simulink library "simulink"  (Simulink 6.0)
settings: Solver=ode45  SolverMode=SingleTasking  StartTime=0.0  StopTime=10.0  RelTol=1e-3
PostLoadFcn:
  | setsysloc(bdroot)
undefined symbols (not defined in the file or in its folder): DiscIntNeverNeededParam, getdatatypespecs, NumBits1, NumBits2, sfunxy, sigbuilder_block, slcm, Slope1, Slope2
libraries: simulink x82, eml_lib x1
(part 3 of 5)

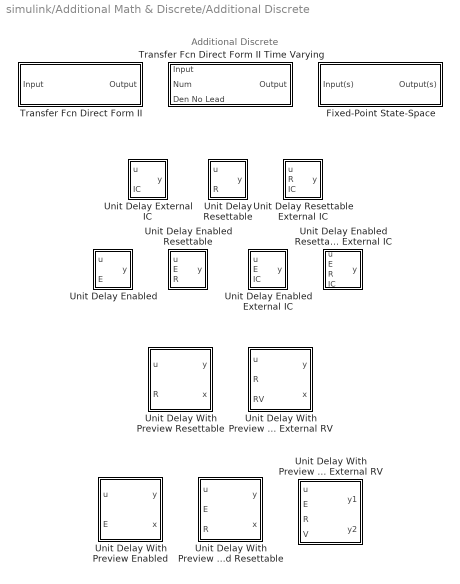
== system simulink/Additional Math & Discrete/Additional Discrete ==
  note: Additional Discrete
  Fixed-Point State-Space : Subsystem  mask(Fixed-Point State-Space){A=[2.6020 -2.2793 0.6708; 1 0 0; 0 1 0], B=[ 1; 0; 0], C=[0.0184    0.0024    0.0055], D=[0.0033], X0=0.0, InternalDataType=float('double'), StateEqScaling=2^0, OutputEqScaling=2^0, LockScale=off, RndMeth=Floor, DoSatur=off}
      mask prompts: A "State Matrix A:"; B "Input Matrix B:"; C "Output Matrix C:"; D "Direct Feedthrough Matrix D:"; X0 "Initial condition for state:"; InternalDataType "Data type for internal calculations:     ex.  sfix(16),  uint(8),  float('single')"; StateEqScaling "Scaling for State Equation AX+BU:   ex.  2^-9"; OutputEqScaling "Scaling for Output Equation CX+DU:   ex.  2^-9"; LockScale "Lock output scaling so autoscaling tool can't change it"; RndMeth "Round toward:"; DoSatur "Saturate to max or min when overflows occur"
      mask help: Discrete-time State-Space Realization
      mask init:
      | blkH = gcbh;
      | blkName = getfullname(blkH);
      | 
      | vRndMeth = get_param(blkH,'RndMeth');
      | vDoSatur = get_param(blkH,'DoSatur');
      | blks = {'State Matrix A','Input Matrix B','Output Matrix C','Direct Link Matrix D','Sum Output Equation','Sum State Equation','Downcast Next State X','Downcast Output Y'};
      | for i = 1:length(blks)
      |   set_param([blkName,'/',blks{i}],'RndMeth',vRndMeth, ...
      | 	  'DoSatur',vDoSatur);
      | end
      mask StyleString: edit,edit,edit,edit,edit,edit,edit,edit,checkbox,popup(Zero|Nearest|Ceiling|Floor),checkbox
      mask TabNameString: Main,Main,Main,Main,Main,Signal data types,Signal data types,Signal data types,Signal data types,Signal data types,Signal data types
      mask Display:
      | text(0.5, 0.5, 'y(n)=Cx(n)+Du(n)', 'horizontalAlignment', 'center', 'verticalAlignment', 'bottom');
      | text(0.5, 0.5, 'x(n+1)=Ax(n)+Bu(n)', 'horizontalAlignment', 'center', 'verticalAlignment', 'top');
  Transfer Fcn Direct Form II : Subsystem  mask(Transfer Fcn Direct Form II){NumCoefVec=[0.2 0.3 0.2], DenCoefVec=[-0.9    0.6], vinit=0.0, RndMeth=Floor, DoSatur=off}
      mask prompts: NumCoefVec "Numerator coefficients:"; DenCoefVec "Denominator coefficients excluding lead (which must be 1.0):"; vinit "Initial condition:"; RndMeth "Round toward:"; DoSatur "Saturate to max or min when overflows occur"
      mask help:
      | A Direct Form II realization of the specified transfer function is used.  Only single input multiple output transfer functions are supported.
      |
      | The data types and scalings of the output, the coefficients, and any temporary variables are automatically selected.  The automatic choices will be acceptable in many situations.  In situations where the automatic choices give unacceptable results, manual layout of the filter is necessary.  For manual layout, it is suggested that the blocks under this mask be used as a starting point.
      |
      | Note 1:
      | The full denominator should have a leading coefficient of +1.0, but this leading coefficient should be excluded when entering the parameter.  For example, if the denominator is
      |   den =
      |             1         -1.7         0.72
      | just enter
      |   den(2:end)  =
      |          -1.7         0.72
      |
      | Note 2:
      | The numerator does NOT need to be the same size as the full denominator.
      mask init:
      | blkH = gcbh;
      | blkName = getfullname(blkH);
      | 
      | vRndMeth = get_param(blkH,'RndMeth');
      | vDoSatur = get_param(blkH,'DoSatur');
      | DCGain = polyval(NumCoefVec,1)./polyval([1 DenCoefVec],1);
      | maxGain = max( 1, max(max(abs(DCGain))) );
      | maxGain = max( maxGain, abs(NumCoefVec(1)) );
      | OutputSlopeMult = 2^ceil(log2(maxGain));
      | DCGain = (1)./polyval([1 DenCoefVec],1);
      | maxGain = max( 1, max(max(abs(DCGain))) );
      | OutputSlopeMult2 = 2^ceil(log2(maxGain));
      | set_param([blkName,'/NumCoef'],'RndMeth',vRndMeth, ...
      | 	'DoSatur',vDoSatur);
      | set_param([blkName,'/DenCoef'],'RndMeth',vRndMeth, ...
      | 	'DoSatur',vDoSatur);
      | set_param([blkName,'/Downcast'],'RndMeth',vRndMeth, ...
      | 	'DoSatur',vDoSatur);
      | set_param([blkName,'/Downcast1'],'RndMeth',vRndMeth, ...
      | 	'DoSatur',vDoSatur);
      | set_param([blkName,'/Sum'],'RndMeth',vRndMeth, ...
      | 	'DoSatur',vDoSatur);
      mask StyleString: edit,edit,edit,popup(Zero|Nearest|Ceiling|Floor),checkbox
      mask Display: dpoly(NumCoefVec,[1 DenCoefVec],'z-')
  Transfer Fcn Direct Form II Time Varying : Subsystem  mask(Transfer Fcn Direct Form II Time Varying){vinit=0.0, RndMeth=Floor, DoSatur=off}
      mask prompts: vinit "Initial condition:"; RndMeth "Round toward:"; DoSatur "Saturate to max or min when overflows occur"
      mask help:
      | A Direct Form II realization of the specified transfer function is used.  Only single input single output transfer functions are supported.
      |
      | The data types and scalings of the output, the coefficients, and any temporary variables are automatically selected.  The automatic choices will be acceptable in many situations.  In situations where the automatic choices give unacceptable results, manual layout of the filter is necessary.  For manual layout, it is suggested that the blocks under this mask be used as a starting point.
      |
      | Note 1:
      | The full denominator should have a leading coefficient of +1.0, but this leading coefficient should be excluded when entering the parameter.  For example, if the denominator is
      |   den =
      |             1         -1.7         0.72
      | just enter
      |   den(2:end)  =
      |          -1.7         0.72
      |
      | Note 2:
      | The numerator does NOT need to be the same size as the full denominator.
      mask init:
      | blkH = gcbh;
      | blkName = getfullname(blkH);
      | 
      | vRndMeth = get_param(blkH,'RndMeth');
      | vDoSatur = get_param(blkH,'DoSatur');
      | set_param([blkName,'/Dot1'],'RndMeth',vRndMeth, ...
      | 	'DoSatur',vDoSatur);
      | set_param([blkName,'/Dot2'],'RndMeth',vRndMeth, ...
      | 	'DoSatur',vDoSatur);
      | set_param([blkName,'/Downcast'],'RndMeth',vRndMeth, ...
      | 	'DoSatur',vDoSatur);
      | set_param([blkName,'/Downcast1'],'RndMeth',vRndMeth, ...
      | 	'DoSatur',vDoSatur);
      | set_param([blkName,'/Sum'],'RndMeth',vRndMeth, ...
      | 	'DoSatur',vDoSatur);
      mask StyleString: edit,popup(Zero|Nearest|Ceiling|Floor),checkbox
      mask Display: fprintf('Direct\nForm II')
  Unit Delay Enabled : Subsystem  mask(Unit Delay Enabled){vinit=0.0, tsamp=-1}
      mask prompts: vinit "Initial condition:"; tsamp "Sample time:"
      mask help:
      | Normally, the output is the signal u delayed by one sample period.
      | When the enable signal is false, the block is disabled, and the state and output values do not change except for resets.  The enable action is vectorized and supports scalar expansion.
      mask Display: dpoly(1,[1 0],'z')
  Unit Delay Enabled External IC : Subsystem  mask(Unit Delay Enabled External Initial Condition){tsamp=-1}
      mask prompts: tsamp "Sample time:"
      mask help:
      | Normally, the output is the signal u delayed by one sample period.
      | The initial condition is given by the signal IC.
      | When the enable signal is false, the block is disabled, and the state and output values do not change except for resets.  The enable action is vectorized and supports scalar expansion.
      mask Display: dpoly(1,[1 0],'z')
  Unit Delay Enabled Resettable : Subsystem  mask(Unit Delay Enabled Resettable){vinit=0.0, tsamp=-1}
      mask prompts: vinit "Initial condition:"; tsamp "Sample time:"
      mask help:
      | Normally, the output is the signal u delayed by one sample period.
      | When the reset signal R is true, the state and the output are always set equal to the initial condition parameter.  This reset action is vectorized and supports scalar expansion.
      | When the enable signal is false, the block is disabled, and the state and output values do not change except for resets.  The enable action is vectorized and supports scalar expansion.
      mask Display: dpoly(1,[1 0],'z')
  Unit Delay Enabled Resettable External IC : Subsystem  mask(Unit Delay Enabled Resettable External Initial Condition){tsamp=-1}
      mask prompts: tsamp "Sample time:"
      mask help:
      | Normally, the output is the signal u delayed by one sample period.
      | When the reset signal R is true, the state and the output are always set equal to the initial condition signal IC.  This reset action is vectorized and supports scalar expansion.
      | When the enable signal is false, the block is disabled, and the state and output values do not change except for resets.  The enable action is vectorized and supports scalar expansion.
      mask Display: dpoly(1,[1 0],'z')
  Unit Delay External IC : Subsystem  mask(Unit Delay External Initial Condition){tsamp=-1}
      mask prompts: tsamp "Sample time:"
      mask help:
      | Normally, the output is the signal u delayed by one sample period.
      | The initial condition is given by the signal IC.
      mask Display: dpoly(1,[1 0],'z')
  Unit Delay Resettable : Subsystem  mask(Unit Delay Resettable){vinit=0.0, tsamp=-1}
      mask prompts: vinit "Initial condition:"; tsamp "Sample time:"
      mask help:
      | Normally, the output is the signal u delayed by one sample period.
      | When the reset signal R is true, the state and the output are always set equal to the initial condition parameter.  This reset action is vectorized and supports scalar expansion.
      mask Display: dpoly(1,[1 0],'z')
  Unit Delay Resettable External IC : Subsystem  mask(Unit Delay Resettable External Initial Condition){tsamp=-1}
      mask prompts: tsamp "Sample time:"
      mask help:
      | Normally, the output is the signal u delayed by one sample period.
      | When the reset signal R is true, the state and the output are always set equal to the initial condition signal IC.  This reset action is vectorized and supports scalar expansion.
      mask Display: dpoly(1,[1 0],'z')
  Unit Delay With Preview Enabled : Subsystem  mask(Unit Delay With Preview Enabled){vinit=0.0, tsamp=-1}
      mask prompts: vinit "Initial condition:"; tsamp "Sample time:"
      mask help:
      | Unit Delays With Preview have two outputs instead of just one.  Normally, the first output equals the signal u, and the second output is a unit delayed version of the first output.
      |
      | Having both signals is useful for implementing recursive calculations where the result should include the most recent inputs.  The second output of a Unit Delay With Preview can be safely fed back into calculations of the block's inputs without causing an algebraic loop.  Meanwhile, the first output will show the most up to date calculations.
      |
      | When the enable signal is false, the block is disabled, and the state and output values do not change except for resets.  The enable action is vectorized and supports scalar expansion.
      mask Display:
      | plot([NaN 0.1 0.13 0.1 NaN 0.1 0.13 0.1 NaN 0.1 0.13 0.1 NaN -0.05 0.025 0.075 0.13 NaN -0.05 0.025 0.075 0.13 NaN 0.13 0.13 0.4475 0.4475 0.13 NaN 0.4475 0.4975 0.5525 0.5225 0.5525 0.5225 NaN 0.4475 0.4975 1.05 NaN 0.5525 0.5525 0.87 0.87 0.5525 NaN 0.71125 0.71125 NaN 0.6525 0.77 NaN 0.6525 0.77 0.6525 0.77 NaN 0.87 0.92 1.05 NaN 0.92 0.92 0.075 0.075 0.13],[NaN 0.846666666666667 0.816666666666667 0.786666666666667 NaN 0.58 0.55 0.52 NaN 0.313333333333333 0.283333333333333 0.253333333333333 NaN 0.75 0.75 0.816666666666667 0.816666666666667 NaN 0.25 0.25 0.55 0.55 NaN 0.15 0.95 0.95 0.15 0.15 NaN 0.55 0.35 0.35 0.38 0.35 0.32 NaN 0.55 0.75 0.75 NaN 0.15 0.55 0.55 0.15 0.15 NaN 0.5 0.4 NaN 0.35 0.35 NaN 0.3 0.3 0.2 0.2 NaN 0.35 0.25 0.25 NaN 0.25 0.05 0.05 0.283333333333333 0.283333333333333]);
      | text(0.23,0.806666666666667,'u');
      | text(0.23,0.54,'E');
  Unit Delay With Preview Enabled Resettable : Subsystem  mask(Unit Delay With Preview Enabled Resettable){vinit=0.0, tsamp=-1}
      mask prompts: vinit "Initial condition:"; tsamp "Sample time:"
      mask help:
      | Unit Delays With Preview have two outputs instead of just one.  Normally, the first output equals the signal u, and the second output is a unit delayed version of the first output.
      |
      | Having both signals is useful for implementing recursive calculations where the result should include the most recent inputs.  The second output of a Unit Delay With Preview can be safely fed back into calculations of the block's inputs without causing an algebraic loop.  Meanwhile, the first output will show the most up to date calculations.
      |
      | The external reset signal R works with the internal initial condition.  When the reset signal R is true, the first output signal is forced to equal the initial condition.  The second output signal is not affected until one time step later.  The internal initial condition is also used to initialize the state when the model starts or when a parent enabled subsystem is reset.  This reset action is vectorized and supports scalar expansion.
      |
      | When the enable signal is false, the block is disabled, and the state and output values do not change except for resets.  The enable action is vectorized and supports scalar expansion.
      mask Display:
      | plot([NaN 0.1 0.13 0.1 NaN 0.1 0.13 0.1 NaN 0.1 0.13 0.1 NaN 0.1 0.13 0.1 NaN -0.05 0.025 0.075 0.13 NaN -0.05 0.025 0.075 0.13 NaN -0.05 0.025 0.075 0.13 NaN 0.13 0.13 0.4475 0.4475 0.13 NaN 0.4475 0.4975 0.5525 0.5225 0.5525 0.5225 NaN 0.4475 0.4975 1.05 NaN 0.5525 0.5525 0.87 0.87 0.5525 NaN 0.71125 0.71125 NaN 0.6525 0.77 NaN 0.6525 0.77 0.6525 0.77 NaN 0.87 0.92 1.05 NaN 0.92 0.92 0.075 0.075 0.13],[NaN 0.88 0.85 0.82 NaN 0.68 0.65 0.62 NaN 0.48 0.45 0.42 NaN 0.28 0.25 0.22 NaN 0.833333333333333 0.833333333333333 0.85 0.85 NaN 0.5 0.5 0.65 0.65 NaN 0.166666666666667 0.166666666666667 0.45 0.45 NaN 0.15 0.95 0.95 0.15 0.15 NaN 0.55 0.35 0.35 0.38 0.35 0.32 NaN 0.55 0.75 0.75 NaN 0.15 0.55 0.55 0.15 0.15 NaN 0.5 0.4 NaN 0.35 0.35 NaN 0.3 0.3 0.2 0.2 NaN 0.35 0.25 0.25 NaN 0.25 0.05 0.05 0.25 0.25]);
      | text(0.23,0.84,'u');
      | text(0.23,0.64,'E');
      | text(0.23,0.44,'R');
  Unit Delay With Preview Enabled Resettable External RV : Subsystem  mask(Unit Delay With Preview Enabled Resettable External RV){vinit=0.0, tsamp=-1}
      mask prompts: vinit "Initial condition:"; tsamp "Sample time:"
      mask help:
      | Unit Delays With Preview have two outputs instead of just one.  Normally, the first output equals the signal u, and the second output is a unit delayed version of the first output.
      |
      | Having both signals is useful for implementing recursive calculations where the result should include the most recent inputs.  The second output of a Unit Delay With Preview can be safely fed back into calculations of the block's inputs without causing an algebraic loop.  Meanwhile, the first output will show the most up to date calculations.
      |
      | This block has both an external reset value and an internal initial condition.  The reset value signal RV is used only when the reset signal R is true.  When this occurs, the first output signal is forced to equal RV.  The second output signal is not affected until one time step later.  The internal initial condition is used only when the model starts or when a parent enabled subsystem is reset.  The internal initial condition only has direct effect on the second output.  The first output is only affected through feedback.  This reset action is vectorized and supports scalar expansion.
      |
      | When the enable signal is false, the block is disabled, and the state and output values do not change except for resets.  The enable action is vectorized and supports scalar expansion.
      mask Display:
      | plot([NaN 0.1 0.13 0.1 NaN 0.1 0.13 0.1 NaN 0.1 0.13 0.1 NaN 0.1 0.13 0.1 NaN 0.1 0.13 0.1 NaN -0.05 0.025 0.075 0.13 NaN -0.05 0.025 0.075 0.13 NaN -0.05 0.025 0.075 0.13 NaN -0.05 0.025 0.075 0.13 NaN 0.13 0.13 0.4475 0.4475 0.13 NaN 0.4475 0.4975 0.5525 0.5225 0.5525 0.5225 NaN 0.4475 0.4975 1.05 NaN 0.5525 0.5525 0.87 0.87 0.5525 NaN 0.71125 0.71125 NaN 0.6525 0.77 NaN 0.6525 0.77 0.6525 0.77 NaN 0.87 0.92 1.05 NaN 0.92 0.92 0.075 0.075 0.13],[NaN 0.9 0.87 0.84 NaN 0.74 0.71 0.68 NaN 0.58 0.55 0.52 NaN 0.42 0.39 0.36 NaN 0.26 0.23 0.2 NaN 0.875 0.875 0.87 0.87 NaN 0.625 0.625 0.71 0.71 NaN 0.375 0.375 0.55 0.55 NaN 0.125 0.125 0.39 0.39 NaN 0.15 0.95 0.95 0.15 0.15 NaN 0.55 0.35 0.35 0.38 0.35 0.32 NaN 0.55 0.75 0.75 NaN 0.15 0.55 0.55 0.15 0.15 NaN 0.5 0.4 NaN 0.35 0.35 NaN 0.3 0.3 0.2 0.2 NaN 0.35 0.25 0.25 NaN 0.25 0.05 0.05 0.23 0.23]);
      | text(0.23,0.86,'u');
      | text(0.23,0.7,'E');
      | text(0.23,0.54,'R');
      | text(0.23,0.38,'RV');
  Unit Delay With Preview Resettable : Subsystem  mask(Unit Delay With Preview Resettable){vinit=0.0, tsamp=-1}
      mask prompts: vinit "Initial condition:"; tsamp "Sample time:"
      mask help:
      | Unit Delays With Preview have two outputs instead of just one.  Normally, the first output equals the signal u, and the second output is a unit delayed version of the first output.
      |
      | Having both signals is useful for implementing recursive calculations where the result should include the most recent inputs.  The second output of a Unit Delay With Preview can be safely fed back into calculations of the block's inputs without causing an algebraic loop.  Meanwhile, the first output will show the most up to date calculations.
      |
      | The external reset signal R works with the internal initial condition.  When the reset signal R is true, the first output signal is forced to equal the initial condition.  The second output signal is not affected until one time step later.  The internal initial condition is also used to initialize the state when the model starts or when a parent enabled subsystem is reset.  This reset action is vectorized and supports scalar expansion.
      mask Display:
      | plot([NaN 0.1 0.13 0.1 NaN 0.1 0.13 0.1 NaN -0.05 0.025 0.075 0.13 NaN -0.05 0.025 0.075 0.13 NaN 0.13 0.13 0.4475 0.4475 0.13 NaN 0.4475 0.4975 0.5525 0.5225 0.5525 0.5225 NaN 0.4475 0.4975 1.05 NaN 0.5525 0.5525 0.87 0.87 0.5525 NaN 0.71125 0.71125 NaN 0.6525 0.77 NaN 0.6525 0.77 0.6525 0.77 NaN 0.87 0.92 1.05],[NaN 0.755 0.725 0.695 NaN 0.305 0.275 0.245 NaN 0.75 0.75 0.725 0.725 NaN 0.25 0.25 0.275 0.275 NaN 0.0499999999999999 0.95 0.95 0.0499999999999999 0.0499999999999999 NaN 0.5 0.275 0.275 0.305 0.275 0.245 NaN 0.5 0.75 0.75 NaN 0.0499999999999999 0.5 0.5 0.0499999999999999 0.0499999999999999 NaN 0.45 0.325 NaN 0.275 0.275 NaN 0.225 0.225 0.0999999999999999 0.0999999999999999 NaN 0.275 0.25 0.25]);
      | text(0.23,0.715,'u');
      | text(0.23,0.265,'R');
  Unit Delay With Preview Resettable External RV : Subsystem  mask(Unit Delay With Preview Resettable External RV){vinit=0.0, tsamp=-1}
      mask prompts: vinit "Initial condition:"; tsamp "Sample time:"
      mask help:
      | Unit Delays With Preview have two outputs instead of just one.  Normally, the first output equals the signal u, and the second output is a unit delayed version of the first output.
      |
      | Having both signals is useful for implementing recursive calculations where the result should include the most recent inputs.  The second output of a Unit Delay With Preview can be safely fed back into calculations of the block's inputs without causing an algebraic loop.  Meanwhile, the first output will show the most up to date calculations.
      |
      | This block has both an external reset value and an internal initial condition.  The reset value signal RV is used only when the reset signal R is true.  When this occurs, the first output signal is forced to equal RV.  The second output signal is not affected until one time step later.  The internal initial condition is used only when the model starts or when a parent enabled subsystem is reset.  The internal initial condition only has direct effect on the second output.  The first output is only affected through feedback.  This reset action is vectorized and supports scalar expansion.
      mask Display:
      | plot([NaN 0.1 0.13 0.1 NaN 0.1 0.13 0.1 NaN 0.1 0.13 0.1 NaN -0.05 0.025 0.075 0.13 NaN -0.05 0.025 0.075 0.13 NaN -0.05 0.025 0.075 0.13 NaN 0.13 0.13 0.4475 0.4475 0.13 NaN 0.4475 0.4975 0.5525 0.5225 0.5525 0.5225 NaN 0.4475 0.4975 1.05 NaN 0.5525 0.5525 0.87 0.87 0.5525 NaN 0.71125 0.71125 NaN 0.6525 0.77 NaN 0.6525 0.77 0.6525 0.77 NaN 0.87 0.92 1.05],[NaN 0.83 0.8 0.77 NaN 0.53 0.5 0.47 NaN 0.23 0.2 0.17 NaN 0.833333333333333 0.833333333333333 0.8 0.8 NaN 0.5 0.5 0.5 0.5 NaN 0.166666666666667 0.166666666666667 0.2 0.2 NaN 0.0499999999999999 0.95 0.95 0.0499999999999999 0.0499999999999999 NaN 0.5 0.275 0.275 0.305 0.275 0.245 NaN 0.5 0.75 0.75 NaN 0.0499999999999999 0.5 0.5 0.0499999999999999 0.0499999999999999 NaN 0.45 0.325 NaN 0.275 0.275 NaN 0.225 0.225 0.0999999999999999 0.0999999999999999 NaN 0.275 0.25 0.25]);
      | text(0.23,0.79,'u');
      | text(0.23,0.49,'R');
      | text(0.23,0.19,'RV');

== system simulink/Additional Math & Discrete/Additional Math: Increment - Decrement ==
  note: Increment/Decrement
  Decrement Real World : Subsystem
      mask Type: Real World Value Decrement
      mask Description:
      | Decrease the Real World Value of Signal by 1.0
      | Overflows will always wrap.
      mask Display: disp('V--')
  Decrement Stored Integer : Subsystem
      mask Type: Stored Integer Value Decrement
      mask Description:
      | Decrease the Stored Value of Signal by 1
      | Floating Point signals are decreased by 1.0
      | Overflows will always wrap.
      mask Display: disp('Q--')
  Decrement To Zero : Subsystem
      mask Type: Decrement To Zero
      mask Description:
      | Decrease the Real World Value of Signal by 1.0,
      | but never go below zero.
      mask Display: fprintf('max( V--, 0 )');
  Decrement Time To Zero : Subsystem
      mask Type: Decrement Time To Zero
      mask Description:
      | Decrease the Real World Value of Signal by the Sample Time Ts,
      | but never go below zero.
      | 
      | This block only works with fixed sample rates, so it will not work inside a triggered subsystem.
      mask Display: fprintf('max( V-Ts, 0 )');
  Increment Real World : Subsystem
      mask Type: Real World Value Increment
      mask Description:
      | Increase the Real World Value of Signal by 1.0
      | Overflows will always wrap.
      mask Display: disp('V++')
  Increment Stored Integer : Subsystem
      mask Type: Stored Integer Value Increment
      mask Description:
      | Increase the Stored Value of Signal by 1
      | Floating Point signals are increased by 1.0
      | Overflows will always wrap.
      mask Display: disp('Q++')

== system simulink/Commonly Used Blocks/Subsystem ==
  In1 : Inport  LatchInput=off
  Out1 : Outport
  wires:
  In1/1 -> Out1/1

== system simulink/Discontinuities/Coulomb & Viscous Friction ==
  In1 : Inport  LatchInput=off
  Gain : Gain  Gain=gain  SaturateOnIntegerOverflow=on
  Gain1 : Gain  Gain=offset  SaturateOnIntegerOverflow=on
  Sign : Signum
  Sum : Sum  Inputs=|++  SaturateOnIntegerOverflow=on  InputSameDT=on
  Out1 : Outport
  wires:
  Sign/1 -> Gain1/1
  In1/1 -> Gain/1, Sign/1
  Gain1/1 -> Sum/1
  Sum/1 -> Out1/1
  Gain/1 -> Sum/2

== system simulink/Discontinuities/Dead Zone Dynamic ==
  up : Inport  LatchInput=off
  u : Inport  Port=2  LatchInput=off
  lo : Inport  Port=3  LatchInput=off
  Diff : Sum  Inputs=+-  OutScaling=2^-10  InputSameDT=on
  Switch : Switch  Criteria=u2 ~= 0  ZeroCross=off  InputSameDT=on
  Switch1 : Switch  Criteria=u2 ~= 0  ZeroCross=off  InputSameDT=on
  u_GTE_up : RelationalOperator  LogicOutDataTypeMode=Boolean  ZeroCross=off
  u_GT_lo : RelationalOperator  Operator=>  LogicOutDataTypeMode=Boolean  ZeroCross=off
  y : Outport
  wires:
  Switch1/1 -> Switch/3
  u/1 -> u_GT_lo/1, Switch1/1, u_GTE_up/1, Diff/1
  u_GT_lo/1 -> Switch1/2
  Diff/1 -> y/1
  Switch/1 -> Diff/2
  lo/1 -> u_GT_lo/2, Switch1/3
  u_GTE_up/1 -> Switch/2
  up/1 -> u_GTE_up/2, Switch/1

== system simulink/Discontinuities/Rate Limiter Dynamic ==
  up : Inport  LatchInput=off
  u : Inport  Port=2  LatchInput=off
  lo : Inport  Port=3  LatchInput=off
  Delay Input2 : UnitDelay  Description=Store in Global RAM  Orientation=left  SampleTime=-1
  Difference Inputs1 : Sum  Description=Add in CPU  Inputs=+-  OutDataType=uint(8)  OutScaling=1
  Difference Inputs2 : Sum  Description=Add in CPU  OutDataType=uint(8)  OutScaling=1
  FixPt Data Type Duplicate : simulink/Signal Attributes/Data Type Duplicate  NumInputPorts=7
  Saturation Dynamic : simulink/Discontinuities/Saturation Dynamic
  delta fall limit : Product  Inputs=**  OutDataType=uint(16)  OutScaling=2^-10  SaturateOnIntegerOverflow=on
  delta rise limit : Product  Inputs=**  OutDataType=uint(16)  OutScaling=2^-10  SaturateOnIntegerOverflow=on
  sample time : simulink/Signal Attributes/Weighted Sample Time  TsampMathOp=Ts Only  weightValue=1  TsampMathImp=Online Calculations  DoSatur=off
  Y : Outport  InitialOutput=0
  wires:
  sample time/1 -> delta rise limit/2, delta fall limit/2
  lo/1 -> delta fall limit/1
  delta rise limit/1 -> Saturation Dynamic/1, FixPt Data Type Duplicate/6
  up/1 -> delta rise limit/1
  Difference Inputs2/1 -> FixPt Data Type Duplicate/1, Delay Input2/1, Y/1  "Y(k)"
  Delay Input2/1 -> FixPt Data Type Duplicate/2, Difference Inputs1/2, Difference Inputs2/2  "Y(k-1)"
  Saturation Dynamic/1 -> FixPt Data Type Duplicate/7, Difference Inputs2/1
  delta fall limit/1 -> Saturation Dynamic/3, FixPt Data Type Duplicate/3
  u/1 -> sample time/1, FixPt Data Type Duplicate/5, Difference Inputs1/1  "U(k)"
  Difference Inputs1/1 -> Saturation Dynamic/2, FixPt Data Type Duplicate/4  "( U(k) - Y(k-1) )"

== system simulink/Discontinuities/Saturation Dynamic ==
  up : Inport  LatchInput=off
  u : Inport  Port=2  LatchInput=off
  lo : Inport  Port=3  LatchInput=off
  Enforce lower limit : MinMax  Function=max  Inputs=2  OutScaling=2^-10  ZeroCross=off
  Enforce upper limit : MinMax  Inputs=2  OutScaling=2^-10  ZeroCross=off
  FixPt Data Type Duplicate : simulink/Signal Attributes/Data Type Duplicate  NumInputPorts=3
  y : Outport
  wires:
  Enforce upper limit/1 -> FixPt Data Type Duplicate/1, y/1
  up/1 -> Enforce upper limit/2
  u/1 -> FixPt Data Type Duplicate/3, Enforce lower limit/2
  Enforce lower limit/1 -> Enforce upper limit/1, FixPt Data Type Duplicate/2
  lo/1 -> Enforce lower limit/1

== system simulink/Discontinuities/Wrap To Zero ==
  U : Inport  LatchInput=off
  FixPt Data Type Duplicate1 : simulink/Signal Attributes/Data Type Duplicate  NumInputPorts=3
  FixPt Switch : Switch  Criteria=u2 > Threshold  Threshold=Threshold  ZeroCross=off
  Ground : Ground
  Y : Outport  InitialOutput=0
  wires:
  Ground/1 -> FixPt Data Type Duplicate1/3, FixPt Switch/1
  FixPt Switch/1 -> Y/1, FixPt Data Type Duplicate1/1
  U/1 -> FixPt Data Type Duplicate1/2, FixPt Switch/3, FixPt Switch/2  "U(k)"

== system simulink/Discrete/Difference ==
  U : Inport  LatchInput=off
  Diff : Sum  Description=Add in CPU  Inputs=+-  OutDataType=OutDataType  OutScaling=OutScaling
  UD : UnitDelay  Description=Store in Global RAM  DisableCoverage=on  X0=ICPrevInput  SampleTime=-1
  Y : Outport  InitialOutput=0
  wires:
  U/1 -> UD/1, Diff/1  "U(k)"
  UD/1 -> Diff/2  "U(k-1)"
  Diff/1 -> Y/1  "( U(k) - U(k-1) )"

== system simulink/Discrete/Discrete Derivative ==
  U : Inport  LatchInput=off
  Data Type Duplicate : simulink/Signal Attributes/Data Type Duplicate  NumInputPorts=3
  Diff : Sum  Description=Add in CPU  Inputs=+-  OutDataType=OutDataType  OutScaling=OutScaling
  TSamp : simulink/Signal Attributes/Weighted Sample Time  TsampMathOp=/  weightValue=1/gainval  TsampMathImp=Offline Scaling Adjustment  DoSatur=off
  UD : UnitDelay  Description=Store in Global RAM  X0=ICPrevScaledInput  SampleTime=-1
  Y : Outport  InitialOutput=0
  wires:
  TSamp/1 -> Data Type Duplicate/2, Diff/1, UD/1
  Diff/1 -> Data Type Duplicate/1, Y/1  "( U(k) - U(k-1) )"
  UD/1 -> Data Type Duplicate/3, Diff/2  "U(k-1)"
  U/1 -> TSamp/1  "U(k)"

== system simulink/Discrete/First-Order Hold ==
  In1 : Inport  LatchInput=off
  Clock : Clock
      settings: DisableCoverage=on  Decimation=10
  Digital Clock : DigitalClock  Orientation=up  DisableCoverage=on  SampleTime=Ts
  Gain : Gain  DisableCoverage=on  Gain=1/Ts  SaturateOnIntegerOverflow=on
  Hit  Crossing : HitCross  DisableCoverage=on  HitCrossingOffset=1  HitCrossingDirection=rising  ShowOutputPort=off
  Output : Sum  Inputs=++|  SaturateOnIntegerOverflow=on  InputSameDT=on
  Product : Product  DisableCoverage=on  SaturateOnIntegerOverflow=on  InputSameDT=on
  Sum : Sum  DisableCoverage=on  Inputs=|+-  SaturateOnIntegerOverflow=on  InputSameDT=on
  Sum2 : Sum  DisableCoverage=on  Inputs=|+-  SaturateOnIntegerOverflow=on  InputSameDT=on
  Unit Delay : UnitDelay  DisableCoverage=on  SampleTime=Ts
  Zero-Order Hold : ZeroOrderHold  DisableCoverage=on  SampleTime=Ts
  Out1 : Outport
  wires:
  Sum/1 -> Product/1
  Unit Delay/1 -> Sum/2
  Product/1 -> Output/2
  Zero-Order Hold/1 -> Output/1, Sum/1
  In1/1 -> Zero-Order Hold/1, Unit Delay/1
  Clock/1 -> Sum2/1
  Digital Clock/1 -> Sum2/2
  Gain/1 -> Hit  Crossing/1, Product/2
  Sum2/1 -> Gain/1
  Output/1 -> Out1/1

== system simulink/Discrete/Transfer Fcn First Order ==
  U : Inport  LatchInput=off
  Data Type Duplicate : simulink/Signal Attributes/Data Type Duplicate  NumInputPorts=3
  Diff : Sum  Description=Add in CPU  Inputs=+-  OutDataType=uint(8)  OutScaling=1
  Gain : Gain  Gain=PoleZ  ParameterDataType=sfix( 16 )  ParameterScalingMode=Best Precision: Column-wise  ParameterScaling=2^-14  OutScaling=2^-10
  Sum : Sum  Description=Add in CPU  OutDataType=sfix(32)  OutScaling=2^-24
  UD : UnitDelay  Description=Store in Global RAM  X0=ICPrevOutput  SampleTime=-1
  Y : Outport  InitialOutput=0
  wires:
  Sum/1 -> Data Type Duplicate/1, UD/1, Y/1  "Y(k)"
  Gain/1 -> Data Type Duplicate/3, Sum/1  "(Pole) ( Y(k-1) - U(k) )"
  Diff/1 -> Gain/1  "( Y(k-1) - U(k) )"
  UD/1 -> Diff/1  "Y(k-1)"
  U/1 -> Data Type Duplicate/2, Sum/2, Diff/2  "U(k)"

== system simulink/Discrete/Transfer Fcn Lead or Lag ==
  Input(s) : Inport  LatchInput=off
  DataTypeProp : simulink/Signal Attributes/Data Type Propagation  PropDataType=sfix(16)  IfRefDouble=double  IfRefSingle=single  IsSigned=IsSigned1 or IsSigned2  NumBitsBase=max([NumBits1 NumBits2])  NumBitsMult=1  NumBitsAdd=0  NumBitsAllowFinal=1:128  PropScaling=2^-10  ValuesUsedBestPrec=[5 -7]  SlopeBase=min([Slope1 Slope2])  SlopeMult=OutputSlopeMult  SlopeAdd=0  BiasBase=Bias1  BiasMult=0  BiasAdd=0
  Delay Input : UnitDelay  Description=Store in Global RAM  X0=ICPrevInput  SampleTime=-1
      settings: AttributesFormatString=%<Description>
  Delay Output : UnitDelay  Description=Store in Global RAM  X0=ICPrevOutput  SampleTime=-1
      settings: AttributesFormatString=%<Description>
  Downcast : DataTypeConversion  Description=|  OutDataType=float('double')  OutScaling=1  LockScale=on
      | Reduce from CPU Size
      |  to Global RAM Size
      settings: AttributesFormatString=%<Description>
  GainPole : Gain  Description=Multiply in CPU  Gain=PoleZ  ParameterDataType=float('double')  ParameterScalingMode=Use specified scaling  ParameterScaling=1  OutDataType=float('double')  OutScaling=1  LockScale=on
      settings: AttributesFormatString=%<Description>
  GainZero : Gain  Description=Multiply in CPU  Gain=ZeroZ  ParameterDataType=float('double')  ParameterScalingMode=Use specified scaling  ParameterScaling=1  OutDataType=float('double')  OutScaling=1  LockScale=on
      settings: AttributesFormatString=%<Description>
  Sum : Sum  Description=Add in CPU  Inputs=+-+  OutDataType=float('double')  OutScaling=1  LockScale=on
      settings: AttributesFormatString=%<Description>
  Output(s) : Outport  InitialOutput=0
  wires:
  Downcast/1 -> DataTypeProp/3, Delay Output/1, Output(s)/1  "Y(k)"
  Sum/1 -> Downcast/1  "(Pole) Y(k-1) + U(k) - (Zero) U(k-1)"
  GainPole/1 -> Sum/3  "(Pole) Y(k-1)"
  GainZero/1 -> Sum/2  "(Zero) U(k-1)"
  Delay Input/1 -> GainZero/1  "U(k-1)"
  Delay Output/1 -> GainPole/1  "Y(k-1)"
  Input(s)/1 -> Delay Input/1, Sum/1, DataTypeProp/1, DataTypeProp/2  "U(k)"

== system simulink/Discrete/Transfer Fcn Real Zero ==
  Input(s) : Inport  LatchInput=off
  DataTypeProp : simulink/Signal Attributes/Data Type Propagation  PropDataType=sfix(16)  IfRefDouble=double  IfRefSingle=single  IsSigned=IsSigned1 or IsSigned2  NumBitsBase=max([NumBits1 NumBits2])  NumBitsMult=1  NumBitsAdd=0  NumBitsAllowFinal=1:128  PropScaling=2^-10  ValuesUsedBestPrec=[5 -7]  SlopeBase=min([Slope1 Slope2])  SlopeMult=OutputSlopeMult  SlopeAdd=0  BiasBase=Bias1  BiasMult=0  BiasAdd=0
  Delay Input : UnitDelay  Description=Store in Global RAM  X0=ICPrevInput  SampleTime=-1
  GainZero : Gain  Description=Multiply in CPU  Gain=ZeroZ  ParameterDataType=float('double')  ParameterScalingMode=Use specified scaling  ParameterScaling=1  OutDataType=float('double')  OutScaling=1  LockScale=on
  Sum : Sum  Description=Add in CPU  Inputs=+-  OutDataType=float('double')  OutScaling=1  LockScale=on
  Output(s) : Outport  InitialOutput=0
  wires:
  Input(s)/1 -> DataTypeProp/2, DataTypeProp/1, Sum/1, Delay Input/1  "U(k)"
  Delay Input/1 -> GainZero/1  "U(k-1)"
  GainZero/1 -> Sum/2  "(Zero) U(k-1)"
  Sum/1 -> Output(s)/1, DataTypeProp/3  "U(k) - (Zero) U(k-1)"

== system simulink/Logic and Bit Operations/Bit Clear ==
  u2 : Inport  LatchInput=off
  Data Type Duplicate : simulink/Signal Attributes/Data Type Duplicate  NumInputPorts=2
  FixPt Bitwise Operator3 : simulink/Logic and Bit Operations/Bitwise Operator  logicop=OR  UseBitMask=on  BitMask=2.^iBit  BitMaskRealWorld=Stored Integer
  FixPt Bitwise Operator4 : simulink/Logic and Bit Operations/Bitwise Operator  logicop=NOT  UseBitMask=off  BitMask=2^iBit  BitMaskRealWorld=Stored Integer
  FixPt Bitwise Operator5 : simulink/Logic and Bit Operations/Bitwise Operator  logicop=NOT  UseBitMask=off  BitMask=2^iBit  BitMaskRealWorld=Stored Integer
  Force To Be Unsigned : DataTypeConversion  OutScaling=2^-10
  Restore Signedness : DataTypeConversion  OutScaling=2^-10
  Same Data Type Except Unsigned : simulink/Signal Attributes/Data Type Propagation  PropDataType=sfix(16)  IfRefDouble=double  IfRefSingle=single  IsSigned=FALSE  NumBitsBase=NumBits1  NumBitsMult=1  NumBitsAdd=0  NumBitsAllowFinal=1:128  PropScaling=2^-10  ValuesUsedBestPrec=[5 -7]  SlopeBase=Slope1  SlopeMult=1  SlopeAdd=0  BiasBase=Bias1  BiasMult=1  BiasAdd=0
  y1 : Outport
  wires:
  Restore Signedness/1 -> Data Type Duplicate/2, y1/1
  Force To Be Unsigned/1 -> Same Data Type Except Unsigned/3, FixPt Bitwise Operator4/1
  u2/1 -> Data Type Duplicate/1, Same Data Type Except Unsigned/2, Same Data Type Except Unsigned/1, Force To Be Unsigned/1
  FixPt Bitwise Operator3/1 -> FixPt Bitwise Operator5/1
  FixPt Bitwise Operator4/1 -> FixPt Bitwise Operator3/1
  FixPt Bitwise Operator5/1 -> Restore Signedness/1

== system simulink/Logic and Bit Operations/Bit Set ==
  u2 : Inport  LatchInput=off
  Data Type Duplicate : simulink/Signal Attributes/Data Type Duplicate  NumInputPorts=2
  FixPt Bitwise Operator1 : simulink/Logic and Bit Operations/Bitwise Operator  logicop=OR  UseBitMask=on  BitMask=2.^iBit  BitMaskRealWorld=Stored Integer
  Force To Be Unsigned : DataTypeConversion  OutScaling=2^-10
  Restore Signedness : DataTypeConversion  OutScaling=2^-10
  Same Data Type Except Unsigned : simulink/Signal Attributes/Data Type Propagation  PropDataType=sfix(16)  IfRefDouble=double  IfRefSingle=single  IsSigned=FALSE  NumBitsBase=NumBits1  NumBitsMult=1  NumBitsAdd=0  NumBitsAllowFinal=1:128  PropScaling=2^-10  ValuesUsedBestPrec=[5 -7]  SlopeBase=Slope1  SlopeMult=1  SlopeAdd=0  BiasBase=Bias1  BiasMult=1  BiasAdd=0
  y1 : Outport
  wires:
  Restore Signedness/1 -> y1/1, Data Type Duplicate/2
  Force To Be Unsigned/1 -> Same Data Type Except Unsigned/3, FixPt Bitwise Operator1/1
  FixPt Bitwise Operator1/1 -> Restore Signedness/1
  u2/1 -> Data Type Duplicate/1, Same Data Type Except Unsigned/2, Same Data Type Except Unsigned/1, Force To Be Unsigned/1

== system simulink/Logic and Bit Operations/Compare To Constant ==
  u : Inport  LatchInput=off
  Compare : RelationalOperator  Operator=<=  LogicOutDataTypeMode=Specify via dialog  ZeroCross=off
  Constant : Constant  Value=const  OutScaling=1
  FixPt Data Type Duplicate : simulink/Signal Attributes/Data Type Duplicate  NumInputPorts=2
  y : Outport
  wires:
  Compare/1 -> y/1
  Constant/1 -> FixPt Data Type Duplicate/2, Compare/2
  u/1 -> FixPt Data Type Duplicate/1, Compare/1

== system simulink/Logic and Bit Operations/Compare To Zero ==
  u : Inport  LatchInput=off
  Compare : RelationalOperator  Operator=<=  LogicOutDataTypeMode=Specify via dialog  ZeroCross=off
  FixPt Data Type Duplicate : simulink/Signal Attributes/Data Type Duplicate  NumInputPorts=2
  Ground : Ground
  y : Outport
  wires:
  Compare/1 -> y/1
  Ground/1 -> FixPt Data Type Duplicate/2, Compare/2
  u/1 -> FixPt Data Type Duplicate/1, Compare/1

== system simulink/Logic and Bit Operations/Detect Change ==
  U : Inport  LatchInput=off
  Delay Input1 : UnitDelay  Description=Store in Global RAM  X0=vinit  SampleTime=-1
  FixPt Relational Operator : RelationalOperator  Operator=~=  LogicOutDataTypeMode=Specify via dialog  ZeroCross=off
  Y : Outport  InitialOutput=0
  wires:
  U/1 -> Delay Input1/1, FixPt Relational Operator/1  "U(k)"
  Delay Input1/1 -> FixPt Relational Operator/2  "U(k-1)"
  FixPt Relational Operator/1 -> Y/1  "Edge"

== system simulink/Logic and Bit Operations/Detect Decrease ==
  U : Inport  LatchInput=off
  Delay Input1 : UnitDelay  Description=Store in Global RAM  X0=vinit  SampleTime=-1
  FixPt Relational Operator : RelationalOperator  Operator=<  LogicOutDataTypeMode=Specify via dialog  ZeroCross=off
  Y : Outport  InitialOutput=0
  wires:
  FixPt Relational Operator/1 -> Y/1  "Edge"
  Delay Input1/1 -> FixPt Relational Operator/2  "U(k-1)"
  U/1 -> FixPt Relational Operator/1, Delay Input1/1  "U(k)"

== system simulink/Logic and Bit Operations/Detect Increase ==
  U : Inport  LatchInput=off
  Delay Input1 : UnitDelay  Description=Store in Global RAM  X0=vinit  SampleTime=-1
  FixPt Relational Operator : RelationalOperator  Operator=>  LogicOutDataTypeMode=Specify via dialog  ZeroCross=off
  Y : Outport  InitialOutput=0
  wires:
  U/1 -> Delay Input1/1, FixPt Relational Operator/1  "U(k)"
  Delay Input1/1 -> FixPt Relational Operator/2  "U(k-1)"
  FixPt Relational Operator/1 -> Y/1  "Edge"

== system simulink/Logic and Bit Operations/Detect Fall Negative ==
  U : Inport  LatchInput=off
  Delay Input1 : UnitDelay  Description=Store in Global RAM  X0=vinit  SampleTime=-1
  FixPt Relational Operator : RelationalOperator  Operator=>  LogicOutDataTypeMode=Specify via dialog  ZeroCross=off
  Negative : simulink/Logic and Bit Operations/Compare To Zero  relop=<  LogicOutDataTypeMode=uint8
  Y : Outport  InitialOutput=0
  wires:
  Negative/1 -> FixPt Relational Operator/1, Delay Input1/1  "U(k)"
  FixPt Relational Operator/1 -> Y/1  "Edge"
  Delay Input1/1 -> FixPt Relational Operator/2  "U(k-1)"
  U/1 -> Negative/1  "U(k)"

== system simulink/Logic and Bit Operations/Detect Fall Nonpositive ==
  U : Inport  LatchInput=off
  Delay Input1 : UnitDelay  Description=Store in Global RAM  X0=vinit  SampleTime=-1
  FixPt Relational Operator : RelationalOperator  Operator=>  LogicOutDataTypeMode=Specify via dialog  ZeroCross=off
  Nonpositive : simulink/Logic and Bit Operations/Compare To Zero  relop=<=  LogicOutDataTypeMode=uint8
  Y : Outport  InitialOutput=0
  wires:
  U/1 -> Nonpositive/1  "U(k)"
  Delay Input1/1 -> FixPt Relational Operator/2  "U(k-1)"
  FixPt Relational Operator/1 -> Y/1  "Edge"
  Nonpositive/1 -> Delay Input1/1, FixPt Relational Operator/1  "U(k)"

== system simulink/Logic and Bit Operations/Detect Rise Nonnegative ==
  U : Inport  LatchInput=off
  Delay Input1 : UnitDelay  Description=Store in Global RAM  X0=vinit  SampleTime=-1
  FixPt Relational Operator : RelationalOperator  Operator=>  LogicOutDataTypeMode=Specify via dialog  ZeroCross=off
  Nonnegative : simulink/Logic and Bit Operations/Compare To Zero  relop=>=  LogicOutDataTypeMode=uint8
  Y : Outport  InitialOutput=0
  wires:
  U/1 -> Nonnegative/1  "U(k)"
  Delay Input1/1 -> FixPt Relational Operator/2  "U(k-1)"
  FixPt Relational Operator/1 -> Y/1  "Edge"
  Nonnegative/1 -> Delay Input1/1, FixPt Relational Operator/1  "U(k)"

== system simulink/Logic and Bit Operations/Detect Rise Positive ==
  U : Inport  LatchInput=off
  Delay Input1 : UnitDelay  Description=Store in Global RAM  X0=vinit  SampleTime=-1
  FixPt Relational Operator : RelationalOperator  Operator=>  LogicOutDataTypeMode=Specify via dialog  ZeroCross=off
  Positive : simulink/Logic and Bit Operations/Compare To Zero  relop=>  LogicOutDataTypeMode=uint8
  Y : Outport  InitialOutput=0
  wires:
  Positive/1 -> FixPt Relational Operator/1, Delay Input1/1  "U(k)"
  FixPt Relational Operator/1 -> Y/1  "Edge"
  Delay Input1/1 -> FixPt Relational Operator/2  "U(k-1)"
  U/1 -> Positive/1  "U(k)"

== system simulink/Logic and Bit Operations/Extract Bits ==
  In : Inport  LatchInput=off
  DTProp1 : simulink/Signal Attributes/Data Type Propagation  PropDataType=sfix(16)  IfRefDouble=double  IfRefSingle=single  IsSigned=IsSigned1  NumBitsBase=NumBits1  NumBitsMult=0.5  NumBitsAdd=0  NumBitsAllowFinal=1:128  PropScaling=2^-10  ValuesUsedBestPrec=[5 -7]  SlopeBase=PosRange1  SlopeMult=2^0  SlopeAdd=0  BiasBase=Bias1  BiasMult=1  BiasAdd=0
  DTProp2 : simulink/Signal Attributes/Data Type Propagation  PropDataType=sfix(16)  IfRefDouble=double  IfRefSingle=single  IsSigned=IsSigned1  NumBitsBase=NumBits1  NumBitsMult=1  NumBitsAdd=0  NumBitsAllowFinal=1:128  PropScaling=1  ValuesUsedBestPrec=[5 -7]  SlopeBase=Slope1  SlopeMult=1  SlopeAdd=0  BiasBase=Bias1  BiasMult=1  BiasAdd=0
  Extract Desired Bits : DataTypeConversion  OutScaling=2^-10
  Modify Scaling Only : DataTypeConversion  OutScaling=2^-10  ConvertRealWorld=Stored Integer (SI)
  Out : Outport
  wires:
  Extract Desired Bits/1 -> DTProp1/3, Modify Scaling Only/1, DTProp2/2, DTProp2/1
  In/1 -> DTProp1/1, DTProp1/2, Extract Desired Bits/1
  Modify Scaling Only/1 -> Out/1, DTProp2/3

== system simulink/Logic and Bit Operations/Interval Test ==
  u : Inport  LatchInput=off
  AND : Logic  AllPortsSameDT=off  OutDataTypeMode=Boolean
  FixPt Data Type Duplicate : simulink/Signal Attributes/Data Type Duplicate  NumInputPorts=3
  Lower Limit : Constant  Value=lowlimit  ConRadixGroup=Best Precision: Vector-wise  OutScaling=2^-1000
  Lower Test : RelationalOperator  Operator=<=  LogicOutDataTypeMode=Specify via dialog  ZeroCross=off
  Upper Limit : Constant  Value=uplimit  ConRadixGroup=Best Precision: Vector-wise  OutScaling=2^-1000
  Upper Test : RelationalOperator  Operator=<=  LogicOutDataTypeMode=Specify via dialog  ZeroCross=off
  y : Outport
  wires:
  Lower Limit/1 -> Lower Test/1, FixPt Data Type Duplicate/2
  Upper Limit/1 -> Upper Test/2, FixPt Data Type Duplicate/3
  Lower Test/1 -> AND/1
  Upper Test/1 -> AND/2
  u/1 -> FixPt Data Type Duplicate/1, Lower Test/2, Upper Test/1
  AND/1 -> y/1

== system simulink/Logic and Bit Operations/Interval Test Dynamic ==
  up : Inport  LatchInput=off
  u : Inport  Port=2  LatchInput=off
  lo : Inport  Port=3  LatchInput=off
  FixPt Data Type Duplicate : simulink/Signal Attributes/Data Type Duplicate  NumInputPorts=3
  FixPt Logical Operator : Logic  AllPortsSameDT=off  OutDataTypeMode=Boolean
  Lower Test : RelationalOperator  Operator=<=  LogicOutDataTypeMode=Specify via dialog  ZeroCross=off
  Upper Test : RelationalOperator  Operator=<=  LogicOutDataTypeMode=Specify via dialog  ZeroCross=off
  y : Outport
  wires:
  FixPt Logical Operator/1 -> y/1
  u/1 -> Lower Test/2, Upper Test/1, FixPt Data Type Duplicate/2
  Upper Test/1 -> FixPt Logical Operator/2
  Lower Test/1 -> FixPt Logical Operator/1
  up/1 -> Upper Test/2, FixPt Data Type Duplicate/3
  lo/1 -> Lower Test/1, FixPt Data Type Duplicate/1

== system simulink/Logic and Bit Operations/Shift Arithmetic ==
  u : Inport  LatchInput=off
  shift : ArithShift  nBitShiftRight=nBitShiftRight  nBinPtShiftRight=nBinPtShiftRight
  y : Outport
  wires:
  u/1 -> shift/1
  shift/1 -> y/1

== system simulink/Lookup Tables/Cosine ==
  In1 : Inport  LatchInput=off
  Handle Quarter Symetery Cosine : Subsystem
      mask Type: Fixed-Point-Private Quandrant Processing Sine
      mask Description:
      | This is a PRIVATE helper block not intended for direct use by customers.
      | This block manages the four possible quandrants that the input signal can be in.  Combining this block with a look up table allows the Sine function to be implemented with 75% less table data.  Only data from the first quandrant is needed.
  Look-Up Table : Lookup  Orientation=left  DialogController=Simulink.DDGSource  InputValues=XData  OutputValues=YData  LookUpMeth=Interpolation-Use End Values  OutDataTypeMode=Specify via dialog  OutScaling=2^-14  LockScale=on
  y : Outport
  wires:
  Handle Quarter Symetery Cosine/2(Input To Lookup Table) -> Look-Up Table/1
  Look-Up Table/1 -> Handle Quarter Symetery Cosine/2(Output From Lookup Table)
  In1/1 -> Handle Quarter Symetery Cosine/1(Raw Angle)
  Handle Quarter Symetery Cosine/1(Cosine) -> y/1

== system simulink/Lookup Tables/Sine ==
  In1 : Inport  LatchInput=off
  Handle Quarter Symetery Sine : Subsystem
      mask Type: Fixed-Point-Private Quandrant Processing Sine
      mask Description:
      | This is a PRIVATE helper block not intended for direct use by customers.
      | This block manages the four possible quandrants that the input signal can be in.  Combining this block with a look up table allows the Sine function to be implemented with 75% less table data.  Only data from the first quandrant is needed.
  Look-Up Table : Lookup  Orientation=left  DialogController=Simulink.DDGSource  InputValues=XData  OutputValues=YData  LookUpMeth=Interpolation-Use End Values  OutDataTypeMode=Specify via dialog  OutScaling=2^-14  LockScale=on
  y : Outport
  wires:
  Handle Quarter Symetery Sine/1(Sine) -> y/1
  In1/1 -> Handle Quarter Symetery Sine/1(Raw Angle)
  Look-Up Table/1 -> Handle Quarter Symetery Sine/2(Output From Lookup Table)
  Handle Quarter Symetery Sine/2(Input To Lookup Table) -> Look-Up Table/1

== system simulink/Math Operations/Algebraic Constraint ==
  f(z) : Inport  LatchInput=off
  Initial Guess : InitialCondition  Value=z0
  Sum : Sum  Inputs=|++  SaturateOnIntegerOverflow=on  InputSameDT=on
  z : Outport
  wires:
  f(z)/1 -> Sum/1
  Initial Guess/1 -> z/1, Sum/2
  Sum/1 -> Initial Guess/1

== system simulink/Math Operations/MinMax Running Resettable ==
  u : Inport  LatchInput=off
  R : Inport  Port=2  LatchInput=off
  Data Type Duplicate : simulink/Signal Attributes/Data Type Duplicate  NumInputPorts=3
  MinMax : MinMax  Inputs=2  OutDataType=uint(8)  OutScaling=1  ZeroCross=off
      settings: LockScale=on
  Unit Delay With Preview Resettable : simulink/Additional Math & Discrete/Additional Discrete/Unit Delay With Preview Resettable  vinit=vinit  tsamp=-1
  y : Outport
  wires:
  Unit Delay With Preview Resettable/1 -> y/1
  MinMax/1 -> Data Type Duplicate/1, Unit Delay With Preview Resettable/1
  Unit Delay With Preview Resettable/2 -> Data Type Duplicate/2, MinMax/2
  u/1 -> Data Type Duplicate/3, MinMax/1
  R/1 -> Unit Delay With Preview Resettable/2  "Reset"

== system simulink/Math Operations/Slider Gain ==
  In1 : Inport  LatchInput=off
  Slider Gain : Gain  Gain=gain  SaturateOnIntegerOverflow=on
  Out1 : Outport
  wires:
  Slider Gain/1 -> Out1/1
  In1/1 -> Slider Gain/1

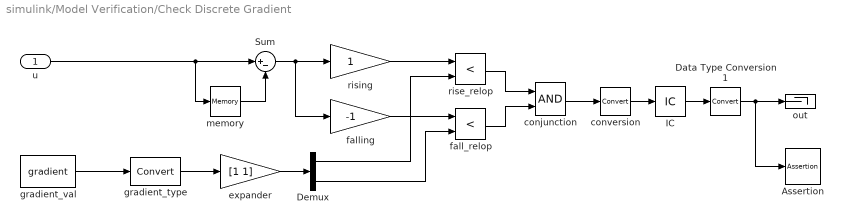
== system simulink/Model Verification/Check Discrete Gradient ==
  u : Inport  LatchInput=off
  Assertion : Assertion
      settings: CopyFcn=set_param(gcbh,'ShadowObject',get_param(get_param(gcbh,'Parent'),'Handle'));
  Data Type Conversion1 : DataTypeConversion  SaturateOnIntegerOverflow=on  RndMeth=Zero
  Demux : Demux  Outputs=2
  IC : InitialCondition
  Sum : Sum  Inputs=|+-  SaturateOnIntegerOverflow=on  InputSameDT=on
  conjunction : Logic
  conversion : DataTypeConversion  SaturateOnIntegerOverflow=on  RndMeth=Zero
  expander : Gain  Gain=[1 1]  SaturateOnIntegerOverflow=on
  fall_relop : RelationalOperator  Operator=<  InputSameDT=on
  falling : Gain  Gain=-1  SaturateOnIntegerOverflow=on
  gradient_type : DataTypeConversion  SaturateOnIntegerOverflow=on  RndMeth=Zero
  gradient_val : Constant  Value=gradient
  memory : Memory  InheritSampleTime=on
  out : Terminator
  rise_relop : RelationalOperator  Operator=<  InputSameDT=on
  rising : Gain  SaturateOnIntegerOverflow=on
  wires:
  Data Type Conversion1/1 -> Assertion/1, out/1
  conversion/1 -> IC/1
  IC/1 -> Data Type Conversion1/1
  conjunction/1 -> conversion/1
  fall_relop/1 -> conjunction/2
  rise_relop/1 -> conjunction/1
  falling/1 -> fall_relop/1
  rising/1 -> rise_relop/1
  Sum/1 -> rising/1, falling/1
  memory/1 -> Sum/2
  Demux/2 -> fall_relop/2
  Demux/1 -> rise_relop/2
  expander/1 -> Demux/1
  u/1 -> Sum/1, memory/1
  gradient_val/1 -> gradient_type/1
  gradient_type/1 -> expander/1
